simulink model "BaseCarroCap4Pag15"  (R2020a)
settings: Solver=ode5  StartTime=0.0  StopTime=200.0  FixedStep=0.05  MaxStep=0.05  RelTol=1e-3
libraries: simulink x1
settings Model: Creator=XICO  LastModifiedBy=XICO
settings SolverCC: InitialStep=200

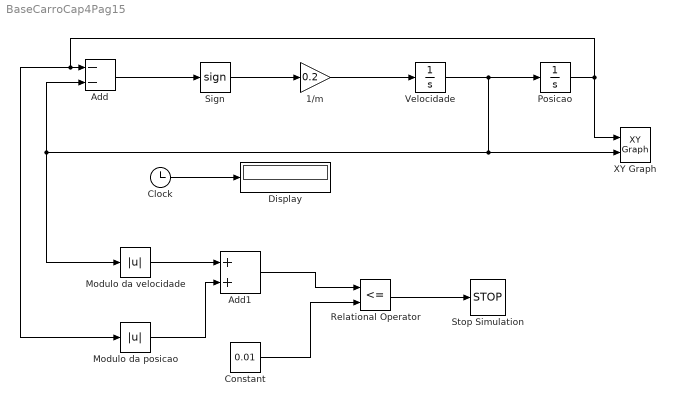
== system BaseCarroCap4Pag15 ==
  1/m : Gain  Gain=0.2
  Add : Sum  Inputs=--
  Add1 : Sum
  Clock : Clock
  Constant : Constant  Value=0.01
  Display : Display
  Modulo da posicao : Abs
  Modulo da velocidade : Abs
  Posicao : Integrator  InitialCondition=1
  Relational Operator : RelationalOperator  Operator=<=  OutDataTypeStr=boolean  RndMeth=Simplest
  Sign : Signum
  Stop Simulation : Stop
  Velocidade : Integrator
  XY Graph : simulink/Sinks/XY Graph  xmin=-1  xmax=1  ymin=-1  ymax=1  st=-1
  wires:
  Posicao/1 -> XY Graph/1, Modulo da posicao/1, Add/1
  Velocidade/1 -> Add/2, Modulo da velocidade/1, XY Graph/2, Posicao/1
  1/m/1 -> Velocidade/1
  Sign/1 -> 1/m/1
  Add/1 -> Sign/1
  Clock/1 -> Display/1
  Relational Operator/1 -> Stop Simulation/1
  Constant/1 -> Relational Operator/2
  Add1/1 -> Relational Operator/1
  Modulo da velocidade/1 -> Add1/1
  Modulo da posicao/1 -> Add1/2
